simulink model "Controlador_PID_final_autosave"  (Simulink 7.7)
settings: Solver=ode45  StartTime=0.0  StopTime=50  RelTol=1e-3
undefined symbols (not defined in the file): bh, bt, bw, Fh0, g, kdx, kdy, kix, kiy, kpx, kpy, Kw, lh_h, lh_min, Mh, mL, Mt, ni, nt, Rd, Rw, Ts, yl0, yt0
libraries: simulink x2
settings Model: Creator=maximiliano  LastModifiedBy=maximiliano

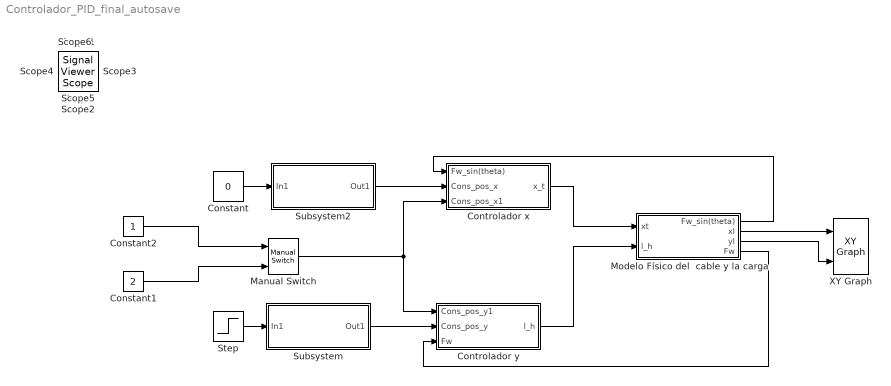
== system Controlador_PID_final_autosave ==
  Constant : Constant  Value=0
  Constant1 : Constant  Value=2
  Constant2 : Constant
  Controlador x : Subsystem
  Controlador y : Subsystem
  Manual Switch : simulink/Signal Routing/Manual Switch  SystemSampleTime=-1  sw=0  action=0  varsize=off
  Modelo Físico del  cable y la carga : Subsystem
  Step : Step  Before=lh_h  After=lh_min  SampleTime=0
  Subsystem : Subsystem
  Subsystem2 : Subsystem
  XY Graph : simulink/Sinks/XY Graph  SystemSampleTime=-1  xmin=-10  xmax=70  ymin=-50  ymax=70  st=-1
  Scope{,1..6} (7 alike) : SignalViewerScope  IOType=viewer  RefreshTime=0.035000
      Scope settings: TimeRange=5  YMin=-2e+270  YMax=1.25e+270
      Scope1 settings: YMin=-1  YMax=1
      Scope2 settings: YMin=-700  YMax=-100  SaveName=ScopeData2
      Scope3 settings: YMin=-1.1  YMax=1.1  SaveName=ScopeData3
      Scope4 settings: SaveName=ScopeData4
      Scope5 settings: YMin=15  YMax=125  SaveName=ScopeData5
      Scope6 settings: YMin=0  YMax=30  SaveName=ScopeData6
  wires:
  Controlador x/1(x_t) -> Modelo Físico del  cable y la carga/1(xt)
  Controlador y/1(l_h) -> Modelo Físico del  cable y la carga/2(l_h)
  Modelo Físico del  cable y la carga/1(Fw_sin(theta)) -> Controlador x/1(Fw_sin(theta))
  Modelo Físico del  cable y la carga/2(xl) -> XY Graph/1
  Modelo Físico del  cable y la carga/3(yl) -> XY Graph/2
  Modelo Físico del  cable y la carga/4(Fw) -> Controlador y/3(Fw)
  Step/1 -> Subsystem/1(In1)
  Subsystem/1(Out1) -> Controlador y/2(Cons_pos_y)
  Constant/1 -> Subsystem2/1(In1)
  Subsystem2/1(Out1) -> Controlador x/2(Cons_pos_x)
  Constant2/1 -> Manual Switch/1
  Constant1/1 -> Manual Switch/2
  Manual Switch/1 -> Controlador x/3(Cons_pos_x1), Controlador y/1(Cons_pos_y1)

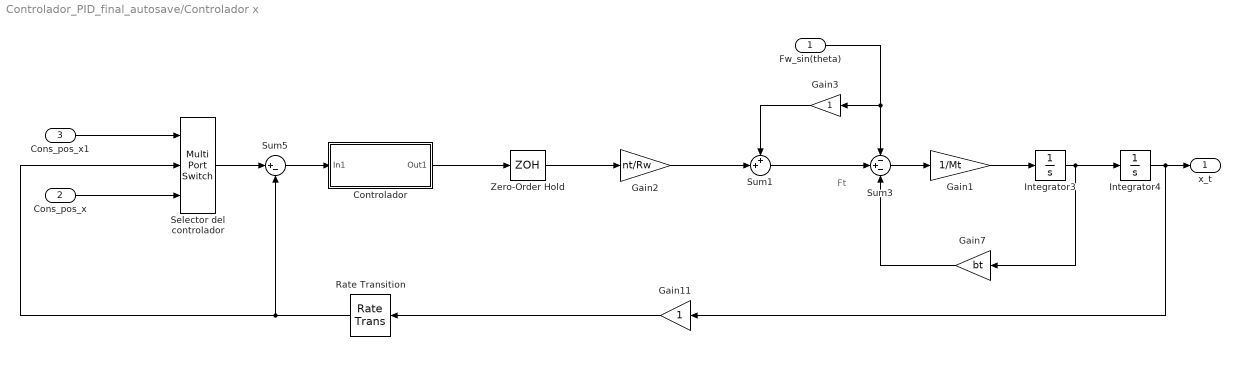
== system Controlador_PID_final_autosave/Controlador x ==
  note: Ft
  Fw_sin(theta) : Inport
  Cons_pos_x : Inport  Port=2
  Cons_pos_x1 : Inport  Port=3
  Controlador : Subsystem
  Gain1 : Gain  Gain=1/Mt
  Gain11 : Gain
  Gain2 : Gain  Gain=nt/Rw
  Gain3 : Gain
  Gain7 : Gain  Gain=bt
  Integrator3 : Integrator
  Integrator4 : Integrator
  Rate Transition : RateTransition  OutPortSampleTime=Ts
  Selector del controlador : MultiPortSwitch  Inputs=2  zeroidx=off
  Sum1 : Sum  Inputs=++|  SampleTime=Ts
  Sum3 : Sum  Inputs=-+-
  Sum5 : Sum  Inputs=|+-
  Zero-Order Hold : ZeroOrderHold  SampleTime=Ts
  x_t : Outport
  wires:
  Gain1/1 -> Integrator3/1
  Integrator3/1 -> Integrator4/1, Gain7/1
  Integrator4/1 -> Gain11/1, x_t/1
  Gain7/1 -> Sum3/3
  Sum3/1 -> Gain1/1
  Gain11/1 -> Rate Transition/1
  Rate Transition/1 -> Sum5/2, Selector del controlador/2
  Zero-Order Hold/1 -> Gain2/1
  Fw_sin(theta)/1 -> Sum3/1, Gain3/1
  Gain3/1 -> Sum1/1
  Selector del controlador/1 -> Sum5/1
  Cons_pos_x1/1 -> Selector del controlador/1
  Cons_pos_x/1 -> Selector del controlador/3
  Sum5/1 -> Controlador/1(In1)
  Controlador/1(Out1) -> Zero-Order Hold/1
  Gain2/1 -> Sum1/2
  Sum1/1 -> Sum3/2

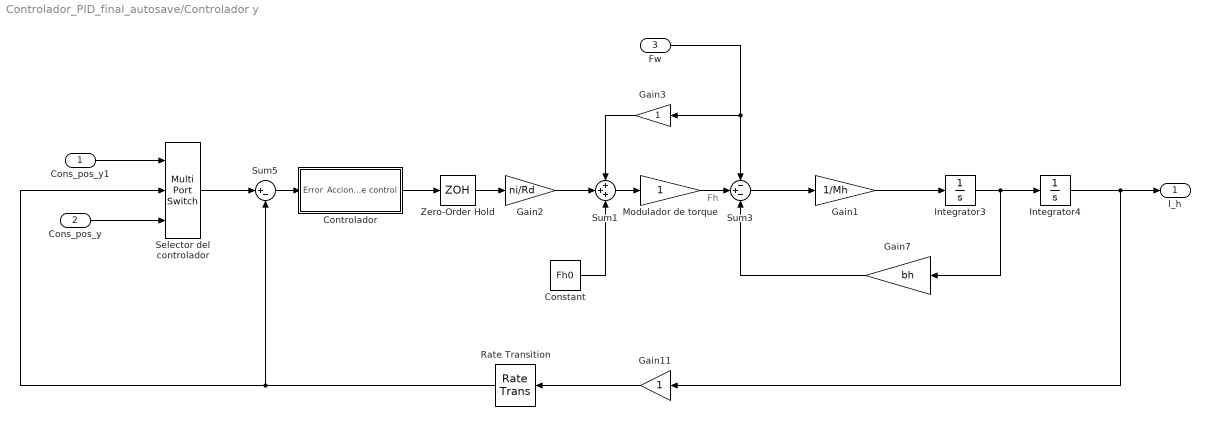
== system Controlador_PID_final_autosave/Controlador y ==
  note: Fh
  Cons_pos_y1 : Inport
  Cons_pos_y : Inport  Port=2
  Fw : Inport  Port=3
  Constant : Constant  Value=Fh0
  Controlador : Subsystem
  Gain1 : Gain  Gain=1/Mh
  Gain11 : Gain
  Gain2 : Gain  Gain=ni/Rd
  Gain3 : Gain
  Gain7 : Gain  Gain=bh
  Integrator3 : Integrator
  Integrator4 : Integrator  InitialCondition=lh_h
  Modulador de torque : Gain
  Rate Transition : RateTransition  OutPortSampleTime=Ts
  Selector del controlador : MultiPortSwitch  Inputs=2  zeroidx=off
  Sum1 : Sum  Inputs=+++
  Sum3 : Sum  Inputs=-+-
  Sum5 : Sum  Inputs=|+-
  Zero-Order Hold : ZeroOrderHold  SampleTime=Ts
  l_h : Outport
  wires:
  Gain1/1 -> Integrator3/1
  Integrator3/1 -> Integrator4/1, Gain7/1
  Integrator4/1 -> l_h/1, Gain11/1
  Gain7/1 -> Sum3/3
  Sum3/1 -> Gain1/1
  Gain11/1 -> Rate Transition/1
  Rate Transition/1 -> Sum5/2, Selector del controlador/2
  Controlador/1(Accion de control) -> Zero-Order Hold/1
  Fw/1 -> Sum3/1, Gain3/1
  Gain3/1 -> Sum1/1
  Selector del controlador/1 -> Sum5/1
  Cons_pos_y1/1 -> Selector del controlador/1
  Cons_pos_y/1 -> Selector del controlador/3
  Sum5/1 -> Controlador/1(Error)
  Zero-Order Hold/1 -> Gain2/1
  Sum1/1 -> Modulador de torque/1
  Modulador de torque/1 -> Sum3/2
  Gain2/1 -> Sum1/2
  Constant/1 -> Sum1/3

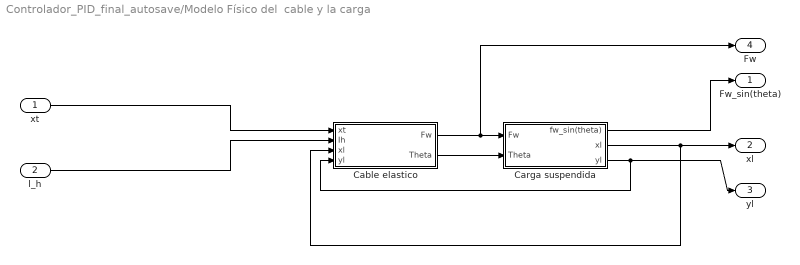
== system Controlador_PID_final_autosave/Modelo Físico del  cable y la carga ==
  xt : Inport
  l_h : Inport  Port=2
  Cable elastico : Subsystem
  Carga suspendida : Subsystem
  Fw_sin(theta) : Outport
  xl : Outport  Port=2
  yl : Outport  Port=3
  Fw : Outport  Port=4
  wires:
  Carga suspendida/3(yl) -> yl/1, Cable elastico/4(yl)
  Carga suspendida/2(xl) -> xl/1, Cable elastico/3(xl)
  xt/1 -> Cable elastico/1(xt)
  l_h/1 -> Cable elastico/2(Ih)
  Carga suspendida/1(fw_sin(theta)) -> Fw_sin(theta)/1
  Cable elastico/1(Fw) -> Carga suspendida/1(Fw), Fw/1
  Cable elastico/2(Theta) -> Carga suspendida/2(Theta)

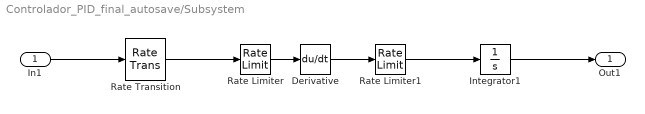
== system Controlador_PID_final_autosave/Subsystem ==
  In1 : Inport
  Derivative : Derivative  LinearizePole=1000
  Integrator1 : Integrator  InitialCondition=lh_h
  Rate Limiter : RateLimiter  RisingSlewLimit=1.5  FallingSlewLimit=-1.5  SampleTimeMode=inherited  InitialCondition=lh_h
  Rate Limiter1 : RateLimiter  SampleTimeMode=inherited
  Rate Transition : RateTransition  OutPortSampleTime=Ts
  Out1 : Outport
  wires:
  Rate Limiter/1 -> Derivative/1
  Derivative/1 -> Rate Limiter1/1
  Rate Limiter1/1 -> Integrator1/1
  Integrator1/1 -> Out1/1
  In1/1 -> Rate Transition/1
  Rate Transition/1 -> Rate Limiter/1

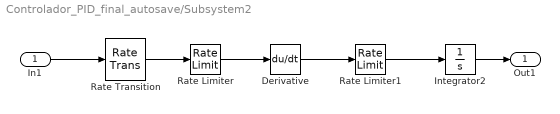
== system Controlador_PID_final_autosave/Subsystem2 ==
  In1 : Inport
  Derivative : Derivative
  Integrator2 : Integrator
  Rate Limiter : RateLimiter  RisingSlewLimit=4  FallingSlewLimit=-4  SampleTimeMode=inherited
  Rate Limiter1 : RateLimiter  RisingSlewLimit=1.5  FallingSlewLimit=-1.5  SampleTimeMode=inherited
  Rate Transition : RateTransition  OutPortSampleTime=Ts
  Out1 : Outport
  wires:
  Rate Limiter/1 -> Derivative/1
  Derivative/1 -> Rate Limiter1/1
  Rate Transition/1 -> Rate Limiter/1
  In1/1 -> Rate Transition/1
  Rate Limiter1/1 -> Integrator2/1
  Integrator2/1 -> Out1/1

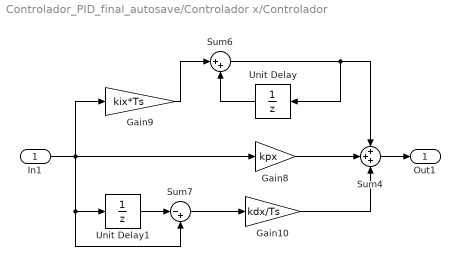
== system Controlador_PID_final_autosave/Controlador x/Controlador ==
  In1 : Inport
  Gain10 : Gain  Gain=kdx/Ts  SampleTime=Ts
  Gain8 : Gain  Gain=kpx  SampleTime=Ts
  Gain9 : Gain  Gain=kix*Ts  SampleTime=Ts
  Sum4 : Sum  Inputs=+++
  Sum6 : Sum  Inputs=|++  SampleTime=Ts
  Sum7 : Sum  Inputs=|-+
  Unit Delay : UnitDelay  SampleTime=Ts
  Unit Delay1 : UnitDelay  SampleTime=Ts
  Out1 : Outport
  wires:
  In1/1 -> Gain8/1, Gain9/1, Unit Delay1/1, Sum7/2
  Gain8/1 -> Sum4/2
  Gain10/1 -> Sum4/3
  Sum6/1 -> Sum4/1, Unit Delay/1
  Unit Delay1/1 -> Sum7/1
  Sum7/1 -> Gain10/1
  Unit Delay/1 -> Sum6/2
  Gain9/1 -> Sum6/1
  Sum4/1 -> Out1/1

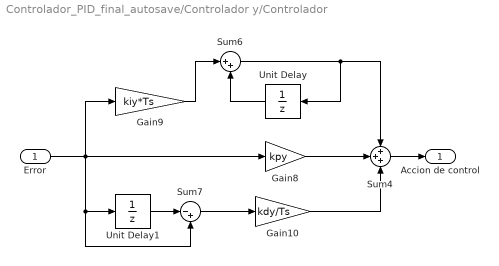
== system Controlador_PID_final_autosave/Controlador y/Controlador ==
  Error : Inport
  Gain10 : Gain  Gain=kdy/Ts  SampleTime=Ts
  Gain8 : Gain  Gain=kpy  SampleTime=Ts
  Gain9 : Gain  Gain=kiy*Ts  SampleTime=Ts
  Sum4 : Sum  Inputs=+++
  Sum6 : Sum  Inputs=|++  SampleTime=Ts
  Sum7 : Sum  Inputs=|-+
  Unit Delay : UnitDelay  SampleTime=Ts
  Unit Delay1 : UnitDelay  SampleTime=Ts
  Accion de control : Outport
  wires:
  Error/1 -> Gain8/1, Gain9/1, Unit Delay1/1, Sum7/2
  Gain8/1 -> Sum4/2
  Gain10/1 -> Sum4/3
  Sum6/1 -> Sum4/1, Unit Delay/1
  Unit Delay1/1 -> Sum7/1
  Sum7/1 -> Gain10/1
  Unit Delay/1 -> Sum6/2
  Gain9/1 -> Sum6/1
  Sum4/1 -> Accion de control/1

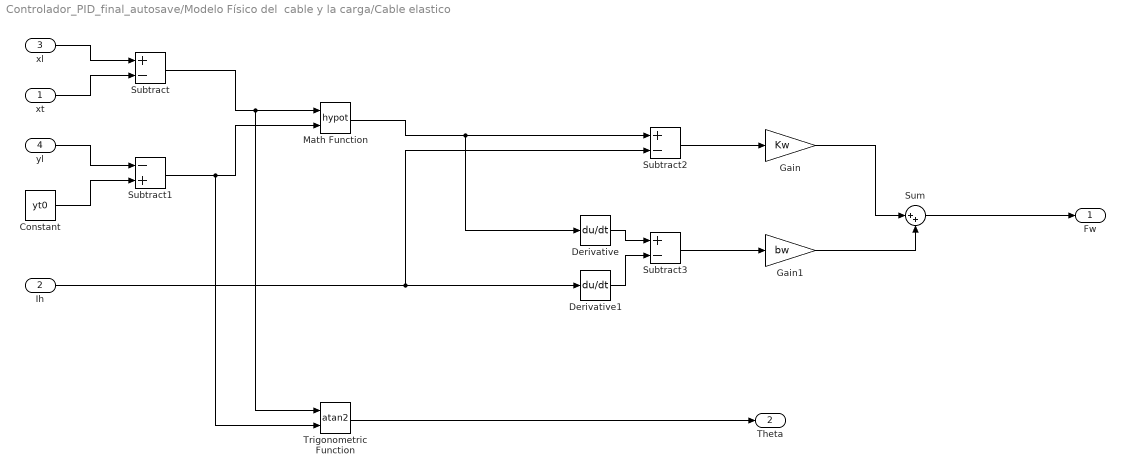
== system Controlador_PID_final_autosave/Modelo Físico del  cable y la carga/Cable elastico ==
  xt : Inport
  Ih : Inport  Port=2
  xl : Inport  Port=3
  yl : Inport  Port=4
  Constant : Constant  Value=yt0
  Derivative : Derivative
  Derivative1 : Derivative
  Gain : Gain  Gain=Kw
  Gain1 : Gain  Gain=bw
  Math Function : Math  Operator=hypot  SaturateOnIntegerOverflow=on
  Subtract : Sum  Inputs=+-
  Subtract1 : Sum  Inputs=-+
  Subtract2 : Sum  Inputs=+-
  Subtract3 : Sum  Inputs=+-
  Sum : Sum  Inputs=|++
  Trigonometric Function : Trigonometry  Operator=atan2
  Fw : Outport
  Theta : Outport  Port=2
  wires:
  xl/1 -> Subtract/1
  xt/1 -> Subtract/2
  Subtract/1 -> Math Function/1, Trigonometric Function/1
  yl/1 -> Subtract1/1
  Constant/1 -> Subtract1/2
  Subtract1/1 -> Math Function/2, Trigonometric Function/2
  Math Function/1 -> Subtract2/1, Derivative/1
  Ih/1 -> Subtract2/2, Derivative1/1
  Subtract2/1 -> Gain/1
  Gain/1 -> Sum/1
  Trigonometric Function/1 -> Theta/1
  Sum/1 -> Fw/1
  Subtract3/1 -> Gain1/1
  Derivative/1 -> Subtract3/1
  Derivative1/1 -> Subtract3/2
  Gain1/1 -> Sum/2

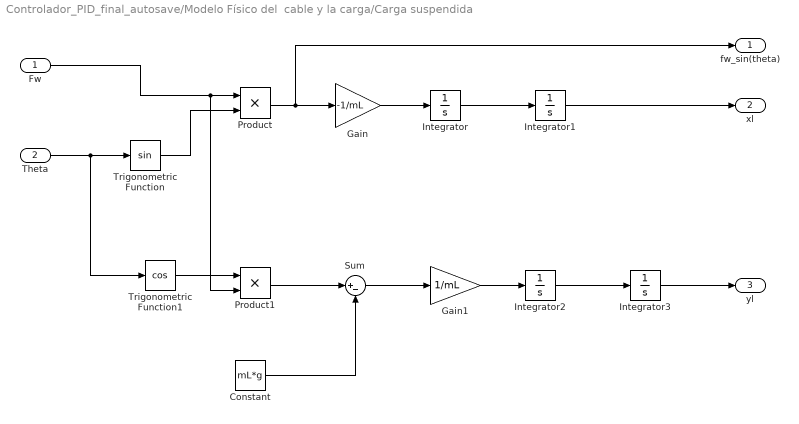
== system Controlador_PID_final_autosave/Modelo Físico del  cable y la carga/Carga suspendida ==
  Fw : Inport
  Theta : Inport  Port=2
  Constant : Constant  Value=mL*g
  Gain : Gain  Gain=-1/mL
  Gain1 : Gain  Gain=1/mL
  Integrator : Integrator
  Integrator1 : Integrator
  Integrator2 : Integrator
  Integrator3 : Integrator  InitialCondition=yl0
  Product : Product  RndMeth=Zero
  Product1 : Product  RndMeth=Zero
  Sum : Sum  Inputs=|+-
  Trigonometric Function : Trigonometry
  Trigonometric Function1 : Trigonometry  Operator=cos
  fw_sin(theta) : Outport
  xl : Outport  Port=2
  yl : Outport  Port=3
  wires:
  Theta/1 -> Trigonometric Function/1, Trigonometric Function1/1
  Fw/1 -> Product/1, Product1/2
  Trigonometric Function/1 -> Product/2
  Product/1 -> Gain/1, fw_sin(theta)/1
  Gain/1 -> Integrator/1
  Integrator/1 -> Integrator1/1
  Integrator1/1 -> xl/1
  Trigonometric Function1/1 -> Product1/1
  Product1/1 -> Sum/1
  Constant/1 -> Sum/2
  Sum/1 -> Gain1/1
  Gain1/1 -> Integrator2/1
  Integrator2/1 -> Integrator3/1
  Integrator3/1 -> yl/1
